simulink model "MIMO_Model_D_R1"  (R2013a)
settings: Solver=ode45  StartTime=0.0  StopTime=sim_length  MaxStep=1e-4  RelTol=1e-3
values from neighbouring files (symbols this model uses):
  A_d = sys_d.a    [MIMO_Controller.m]
  B_d = sys_d.b    [MIMO_Controller.m]
  C_d = sys_d.c    [MIMO_Controller.m]
  G_MIMO_d = place(A_d',C_d',P)'    [MIMO_Controller.m]
  K_MIMO_d = K_MIMO_Reg    [MIMO_Controller.m]
  omega_0 = 500    [MIMO_Controller.m]
  omega_Lim = -inf*(0-F_yIntercept)/Kf    [MIMO_Controller.m]
  Phi_IC = (0/180)*pi    (= 0)    [MIMO_Controller.m]
  Pitch_Setpoint = 0    [MIMO_Controller.m]
  Psi_IC = (0/180)*pi    (= 0)    [MIMO_Controller.m]
  PWM_LimHigher = 2*inf    (= inf)    [MIMO_Controller.m]
  PWM_LimLower = 1.1*-inf    (= -inf)    [MIMO_Controller.m]
  Theta_IC = (5/180)*pi    (= 0.0872664625997)    [MIMO_Controller.m]
  Ts = 30e-3    (= 0.03)    [MIMO_Controller.m]
  Yaw_Setpoint = 0    [MIMO_Controller.m]
undefined symbols (not defined in the file or in its folder): Drag, F_yIntercept, g, I_Phi, I_Psi, I_Theta, J, Kf, Kw, L, Mass, Motor_TimeConstant, Speed_yIntercept
libraries: simulink x6
settings Model: Creator=Ross  LastModifiedBy=Ross

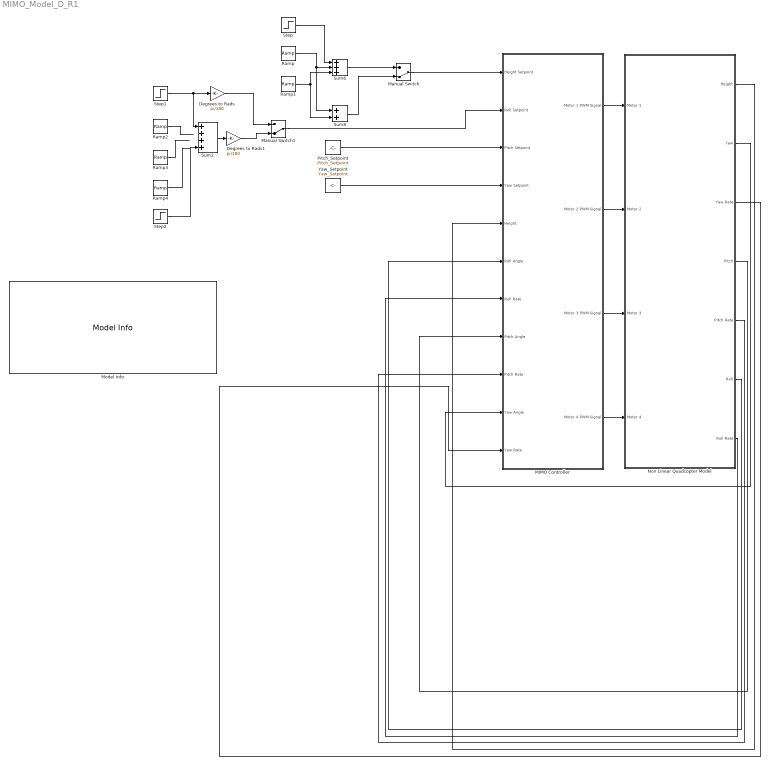
== system MIMO_Model_D_R1 ==
  Degrees to Rads : Gain  Gain=pi/180
  Degrees to Rads1 : Gain  Gain=pi/180
  MIMO Controller : Subsystem
  Manual Switch : ManualSwitch  CurrentSetting=0
  Manual Switch1 : ManualSwitch  CurrentSetting=0
  Model Info : simulink/Model-Wide Utilities/Model Info  InitialBlockCM=None  BlockCM=None  Frame=on  DisplayStringWithTags=|  HorizontalTextAlignment=Center  LeftAlignmentValue=0.5  SourceBlockDiagram=MIMO_Model_D_R1  TagMaxNumber=20
      | %<ModelName>
      | Simulink Diagram Used in Testing of Controllers designed for Quadcopters
      | Model version is %<ModelVersion>
      | 
      | %<Created>
      | %<ModifiedBy>
      | %<ModifiedDate>
      | %<ModifiedComment>
      | 
      | 
      | %<LastModifiedBy>
      | %<LastModificationDate>
      | %<Description>
  Non Linear Quadcopter Model : Subsystem
  "Pitch_Setpoint " : Constant  Value=Pitch_Setpoint
  Ramp : simulink/Sources/Ramp  slope=1  start=2  X0=0
  Ramp1 : simulink/Sources/Ramp  slope=-1  start=5  X0=0
  Ramp2 : simulink/Sources/Ramp  slope=10  start=2  X0=Ts
  Ramp3 : simulink/Sources/Ramp  slope=-20  start=4  X0=Ts
  Ramp4 : simulink/Sources/Ramp  slope=10  start=6  X0=Ts
  Step : Step  Time=10  SampleTime=0
  Step1 : Step  Time=2  After=20  SampleTime=Ts
  Step2 : Step  Time=4  After=-20  SampleTime=Ts
  Sum2 : Sum  Inputs=++++
  Sum6 : Sum  Inputs=+++  SampleTime=Ts
  Sum8 : Sum  SampleTime=Ts
  Yaw_Setpoint : Constant  Value=Yaw_Setpoint
  wires:
  Non Linear Quadcopter Model/1(Height) -> MIMO Controller/5(Height)
  Non Linear Quadcopter Model/5(Pitch Rate) -> MIMO Controller/9(Pitch Rate)
  Non Linear Quadcopter Model/7(Roll Rate) -> MIMO Controller/7(Roll Rate)
  Ramp/1 -> Sum8/1, Sum6/2
  Ramp1/1 -> Sum8/2, Sum6/3
  Step/1 -> Sum6/1
  Manual Switch/1 -> MIMO Controller/1(Height Setpoint)
  Sum8/1 -> Manual Switch/2
  Sum6/1 -> Manual Switch/1
  Non Linear Quadcopter Model/6(Roll) -> MIMO Controller/6(Roll Angle)
  Non Linear Quadcopter Model/4(Pitch) -> MIMO Controller/8(Pitch Angle)
  Ramp2/1 -> ?
  Ramp3/1 -> ?
  Step1/1 -> Sum2/1, Degrees to Rads/1
  Sum2/1 -> Degrees to Rads1/1
  Degrees to Rads/1 -> Manual Switch1/1
  "Pitch_Setpoint "/1 -> MIMO Controller/3(Pitch Setpoint)
  Manual Switch1/1 -> MIMO Controller/2(Roll Setpoint)
  Yaw_Setpoint/1 -> MIMO Controller/4(Yaw Setpoint)
  MIMO Controller/3(Motor 3 PWM Signal) -> Non Linear Quadcopter Model/3(Motor 3)
  MIMO Controller/2(Motor 2 PWM Signal) -> Non Linear Quadcopter Model/2(Motor 2)
  MIMO Controller/1(Motor 1 PWM Signal) -> Non Linear Quadcopter Model/1(Motor 1)
  Degrees to Rads1/1 -> Manual Switch1/2
  Step2/1 -> Sum2/4
  Ramp4/1 -> ?
  MIMO Controller/4(Motor 4 PWM Signal) -> Non Linear Quadcopter Model/4(Motor 4)
  Non Linear Quadcopter Model/2(Yaw) -> MIMO Controller/10(Yaw Angle)
  Non Linear Quadcopter Model/3(Yaw Rate) -> MIMO Controller/11(Yaw Rate)

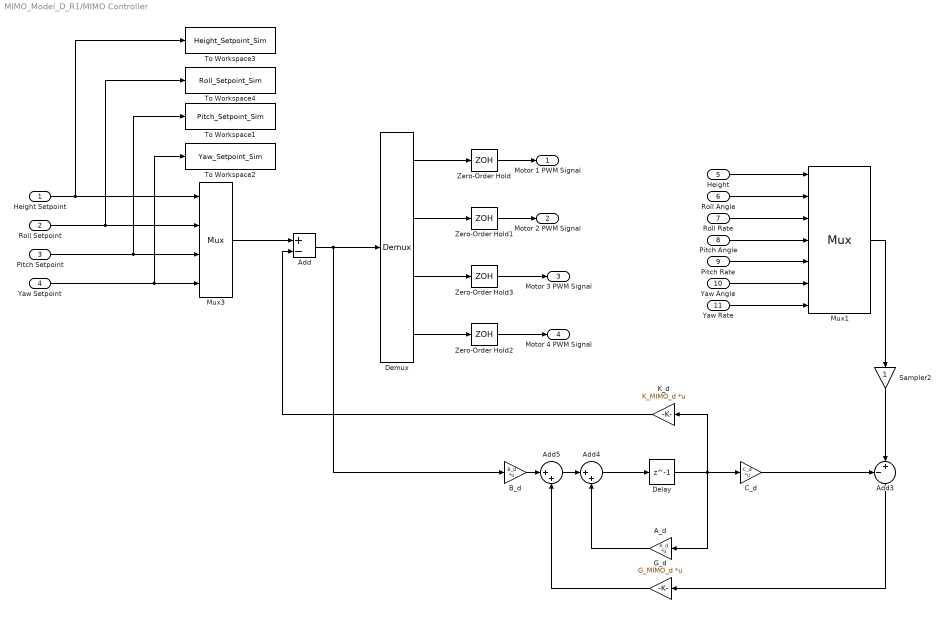
== system MIMO_Model_D_R1/MIMO Controller ==
  Height Setpoint : Inport
  Roll Setpoint : Inport  Port=2
  Pitch Setpoint : Inport  Port=3
  Yaw Setpoint : Inport  Port=4
  Height : Inport  Port=5
  Roll Angle : Inport  Port=6
  Roll Rate : Inport  Port=7
  Pitch Angle : Inport  Port=8
  Pitch Rate : Inport  Port=9
  Yaw Angle : Inport  Port=10
  Yaw Rate : Inport  Port=11
  A_d : Gain  Gain=A_d  Multiplication=Matrix(K*u)  SampleTime=Ts
  Add : Sum  Inputs=+-  SampleTime=Ts
  Add3 : Sum  Inputs=-+|
  Add4 : Sum  Inputs=|++
  Add5 : Sum  Inputs=|++
  "B_d " : Gain  Gain=B_d  Multiplication=Matrix(K*u)  SampleTime=Ts
  "C_d " : Gain  Gain=C_d  Multiplication=Matrix(K*u)  SampleTime=Ts
  Delay : Delay  DelayLength=1  InitialCondition=0  SampleTime=Ts
  Demux : Demux
  G_d : Gain  Gain=G_MIMO_d  Multiplication=Matrix(K*u)  SampleTime=Ts
  K_d : Gain  Gain=K_MIMO_d  Multiplication=Matrix(K*u)  SampleTime=Ts
  Mux1 : Mux  Inputs=7
      settings: DisplayOption=signals
  Mux3 : Mux
      settings: DisplayOption=signals
  Sampler2 : Gain  SampleTime=Ts
  To Workspace1 : ToWorkspace  VariableName=Pitch_Setpoint_Sim  SampleTime=-1  SaveFormat=Timeseries
  To Workspace2 : ToWorkspace  VariableName=Yaw_Setpoint_Sim  SampleTime=-1  SaveFormat=Timeseries
  To Workspace3 : ToWorkspace  VariableName=Height_Setpoint_Sim  SampleTime=-1  SaveFormat=Timeseries
  To Workspace4 : ToWorkspace  VariableName=Roll_Setpoint_Sim  SampleTime=-1  SaveFormat=Timeseries
  Zero-Order Hold{,1..3} (4 alike) : ZeroOrderHold  SampleTime=Ts
  Motor 1 PWM Signal : Outport
  Motor 2 PWM Signal : Outport  Port=2
  Motor 3 PWM Signal : Outport  Port=3
  Motor 4 PWM Signal : Outport  Port=4
  wires:
  Roll Angle/1 -> Mux1/2
  Height/1 -> Mux1/1
  Add5/1 -> Add4/1
  Mux1/1 -> Sampler2/1
  G_d/1 -> Add5/2
  A_d/1 -> Add4/2
  Add4/1 -> Delay/1
  "C_d "/1 -> Add3/1
  K_d/1 -> Add/2
  Sampler2/1 -> Add3/2
  "B_d "/1 -> Add5/1
  Delay/1 -> K_d/1, "C_d "/1, A_d/1
  Add3/1 -> G_d/1
  Add/1 -> "B_d "/1, Demux/1
  Roll Rate/1 -> Mux1/3
  Pitch Angle/1 -> Mux1/4
  Pitch Rate/1 -> Mux1/5
  Yaw Angle/1 -> Mux1/6
  Yaw Rate/1 -> Mux1/7
  Height Setpoint/1 -> To Workspace3/1, Mux3/1
  Roll Setpoint/1 -> To Workspace4/1, Mux3/2
  Pitch Setpoint/1 -> To Workspace1/1, Mux3/3
  Yaw Setpoint/1 -> To Workspace2/1, Mux3/4
  Mux3/1 -> Add/1
  Demux/1 -> Zero-Order Hold/1
  Demux/2 -> Zero-Order Hold1/1
  Demux/3 -> Zero-Order Hold3/1
  Demux/4 -> Zero-Order Hold2/1
  Zero-Order Hold/1 -> Motor 1 PWM Signal/1
  Zero-Order Hold1/1 -> Motor 2 PWM Signal/1
  Zero-Order Hold3/1 -> Motor 3 PWM Signal/1
  Zero-Order Hold2/1 -> Motor 4 PWM Signal/1

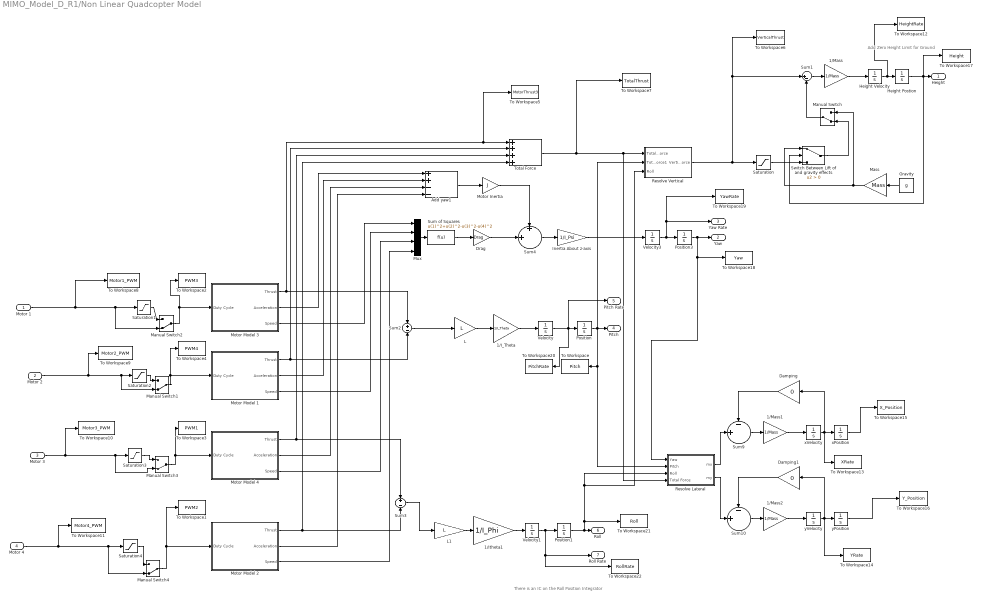
== system MIMO_Model_D_R1/Non Linear Quadcopter Model ==
  note: There is an IC on the Roll
      | Position Integrator
  note: Add Zero Height Limit
      | for Ground
  Motor 1 : Inport
  Motor 2 : Inport  Port=2
  Motor 3 : Inport  Port=3
  Motor 4 : Inport  Port=4
  1/I_Theta : Gain  Gain=1/I_Theta
  1/Itheta1 : Gain  Gain=1/I_Phi
  1/Mass : Gain  Gain=1/Mass
  1/Mass1 : Gain  Gain=1/Mass
  1/Mass2 : Gain  Gain=1/Mass
  Add yaw1 : Sum  Inputs=++--
  Damping : Gain  Gain=0
  Damping1 : Gain  Gain=0
  Drag : Gain  Gain=Drag
  Gravity : Constant  Value=g
  Height Postion : Integrator  LowerSaturationLimit=0
  Height Velocity : Integrator
  Inertia About z-axis : Gain  Gain=1/I_Psi
  L : Gain  Gain=L
  L1 : Gain  Gain=L
  Manual Switch{,1..4} (5 alike) : ManualSwitch  CurrentSetting=0
  Mass : Gain  Gain=Mass
  Motor Inertia : Gain  Gain=J
  Motor Model 1 : Subsystem
  Motor Model 2 : Subsystem
  Motor Model 3 : Subsystem
  Motor Model 4 : Subsystem
  Mux : Mux
  Position : Integrator  InitialCondition=Theta_IC
  Position1 : Integrator  InitialCondition=Phi_IC
  Position3 : Integrator  InitialCondition=Psi_IC
  Resolve Lateral : Subsystem
  Resolve Vertical : Subsystem
  Saturation : Saturate  UpperLimit=Mass*g  LowerLimit=-inf
  Saturation{1..4} (4 alike) : Saturate  UpperLimit=PWM_LimHigher  LowerLimit=PWM_LimLower
  Sum of Squares : Fcn  Expr=u(1)^2+u(2)^2-u(3)^2-u(4)^2
  Sum1 : Sum  Inputs=|+-
  Sum10 : Sum  Inputs=-|||+||||
  Sum2 : Sum  Inputs=+|-
  Sum3 : Sum  Inputs=+|-
  Sum4 : Sum  Inputs=+|||+||||
  Sum9 : Sum  Inputs=-|||+||||
  Switch Between Lift of and gravity effects : Switch  Criteria=u2 > Threshold
  To Workspace : ToWorkspace  VariableName=Pitch  SampleTime=-1  SaveFormat=Timeseries
  To Workspace1 : ToWorkspace  VariableName=PWM2  SampleTime=-1  SaveFormat=Timeseries
  To Workspace10 : ToWorkspace  VariableName=Motor3_PWM  SampleTime=-1  SaveFormat=Timeseries
  To Workspace11 : ToWorkspace  VariableName=Motor4_PWM  SampleTime=-1  SaveFormat=Timeseries
  To Workspace12 : ToWorkspace  VariableName=HeightRate  SampleTime=-1  SaveFormat=Timeseries
  To Workspace13 : ToWorkspace  VariableName=XRate  SampleTime=-1  SaveFormat=Timeseries
  To Workspace14 : ToWorkspace  VariableName=YRate  SampleTime=-1  SaveFormat=Timeseries
  To Workspace15 : ToWorkspace  VariableName=X_Position  SampleTime=-1  SaveFormat=Timeseries
  To Workspace16 : ToWorkspace  VariableName=Y_Position  SampleTime=-1  SaveFormat=Timeseries
  To Workspace17 : ToWorkspace  VariableName=Height  SampleTime=-1  SaveFormat=Timeseries
  To Workspace18 : ToWorkspace  VariableName=Yaw  SampleTime=-1  SaveFormat=Timeseries
  To Workspace19 : ToWorkspace  VariableName=YawRate  SampleTime=-1  SaveFormat=Timeseries
  To Workspace2 : ToWorkspace  VariableName=PWM3  SampleTime=-1  SaveFormat=Timeseries
  To Workspace20 : ToWorkspace  VariableName=PitchRate  SampleTime=-1  SaveFormat=Timeseries
  To Workspace21 : ToWorkspace  VariableName=Roll  SampleTime=-1  SaveFormat=Timeseries
  To Workspace22 : ToWorkspace  VariableName=RollRate  SampleTime=-1  SaveFormat=Timeseries
  To Workspace3 : ToWorkspace  VariableName=PWM1  SampleTime=-1  SaveFormat=Timeseries
  To Workspace4 : ToWorkspace  VariableName=PWM4  SampleTime=-1  SaveFormat=Timeseries
  To Workspace5 : ToWorkspace  VariableName=MotorThrust3  SampleTime=-1  SaveFormat=Timeseries
  To Workspace6 : ToWorkspace  VariableName=VerticalThrust  SampleTime=-1  SaveFormat=Timeseries
  To Workspace7 : ToWorkspace  VariableName=TotalThrust  SampleTime=-1  SaveFormat=Timeseries
  To Workspace8 : ToWorkspace  VariableName=Motor1_PWM  SampleTime=-1  SaveFormat=Timeseries
  To Workspace9 : ToWorkspace  VariableName=Motor2_PWM  SampleTime=-1  SaveFormat=Timeseries
  Total Force : Sum  Inputs=++++
  Velocity : Integrator
  Velocity1 : Integrator
  Velocity3 : Integrator
  xPosition : Integrator
  xVelocity : Integrator
  yPosition : Integrator
  yVelocity : Integrator
  Height : Outport
  Yaw : Outport  Port=2
  Yaw Rate : Outport  Port=3
  Pitch : Outport  Port=4
  Pitch Rate : Outport  Port=5
  Roll : Outport  Port=6
  Roll Rate : Outport  Port=7
  wires:
  Sum1/1 -> 1/Mass/1
  Motor 3/1 -> Manual Switch3/2, Saturation3/1, To Workspace10/1
  Add yaw1/1 -> Motor Inertia/1
  1/Mass/1 -> Height Velocity/1
  Motor Inertia/1 -> Sum4/1
  1/Mass1/1 -> xVelocity/1
  Sum9/1 -> 1/Mass1/1
  xPosition/1 -> To Workspace15/1
  Damping/1 -> Sum9/1
  xVelocity/1 -> To Workspace13/1, Damping/1, xPosition/1
  Motor Model 3/2(Acceleration) -> Add yaw1/1
  Height Velocity/1 -> To Workspace12/1, Height Postion/1
  Sum2/1 -> L/1
  1/I_Theta/1 -> Velocity/1
  Velocity/1 -> To Workspace20/1, Pitch Rate/1, Position/1
  Position/1 -> Resolve Vertical/2(Total Force1), Pitch/1, To Workspace/1, Resolve Lateral/2(Pitch)
  Total Force/1 -> To Workspace7/1, Resolve Lateral/4(Total Force), Resolve Vertical/1(Total Force)
  Sum of Squares/1 -> Drag/1
  Drag/1 -> Sum4/2
  Position3/1 -> To Workspace18/1, Resolve Lateral/1(Yaw), Yaw/1
  Velocity3/1 -> To Workspace19/1, Yaw Rate/1, Position3/1
  Inertia About z-axis/1 -> Velocity3/1
  Motor Model 2/1(Thrust) -> Total Force/4, Sum3/2
  L1/1 -> 1/Itheta1/1
  Velocity1/1 -> To Workspace22/1, Roll Rate/1, Position1/1
  Sum3/1 -> L1/1
  Position1/1 -> Roll/1, To Workspace21/1, Resolve Lateral/3(Roll), Resolve Vertical/3(Roll)
  1/Itheta1/1 -> Velocity1/1
  Motor Model 3/1(Thrust) -> To Workspace5/1, Total Force/1, Sum2/1
  Sum10/1 -> 1/Mass2/1
  1/Mass2/1 -> yVelocity/1
  Damping1/1 -> Sum10/1
  yVelocity/1 -> Damping1/1, To Workspace14/1, yPosition/1
  Height Postion/1 -> Switch Between Lift of and gravity effects/2, To Workspace17/1, Height/1
  Motor Model 4/2(Acceleration) -> Add yaw1/3
  Motor Model 1/1(Thrust) -> Total Force/2, Sum2/2
  Sum4/1 -> Inertia About z-axis/1
  Motor Model 4/1(Thrust) -> Total Force/3, Sum3/1
  Motor 1/1 -> To Workspace8/1, Manual Switch2/2, Saturation1/1
  Motor 2/1 -> Manual Switch1/2, Saturation2/1, To Workspace9/1
  Motor Model 1/2(Acceleration) -> Add yaw1/2
  Motor Model 2/2(Acceleration) -> Add yaw1/4
  Motor 4/1 -> Manual Switch4/2, Saturation4/1, To Workspace11/1
  Gravity/1 -> Mass/1
  Resolve Lateral/1(mx) -> Sum9/2
  Resolve Lateral/2(my) -> Sum10/2
  Motor Model 3/3(Speed) -> Mux/1
  Motor Model 1/3(Speed) -> Mux/2
  Motor Model 4/3(Speed) -> Mux/3
  Motor Model 2/3(Speed) -> Mux/4
  Mux/1 -> Sum of Squares/1
  L/1 -> 1/I_Theta/1
  Switch Between Lift of and gravity effects/1 -> Manual Switch/2
  Saturation/1 -> Switch Between Lift of and gravity effects/3
  Mass/1 -> Manual Switch/1, Switch Between Lift of and gravity effects/1
  Manual Switch/1 -> Sum1/2
  Resolve Vertical/1(Vertical Force) -> Sum1/1, To Workspace6/1, Saturation/1
  yPosition/1 -> To Workspace16/1
  Manual Switch2/1 -> To Workspace2/1, Motor Model 3/1(Duty Cycle)
  Manual Switch1/1 -> To Workspace4/1, Motor Model 1/1(Duty Cycle)
  Manual Switch3/1 -> Motor Model 4/1(Duty Cycle), To Workspace3/1
  Manual Switch4/1 -> To Workspace1/1, Motor Model 2/1(Duty Cycle)
  Saturation2/1 -> Manual Switch1/1
  Saturation4/1 -> Manual Switch4/1
  Saturation3/1 -> Manual Switch3/1
  Saturation1/1 -> Manual Switch2/1

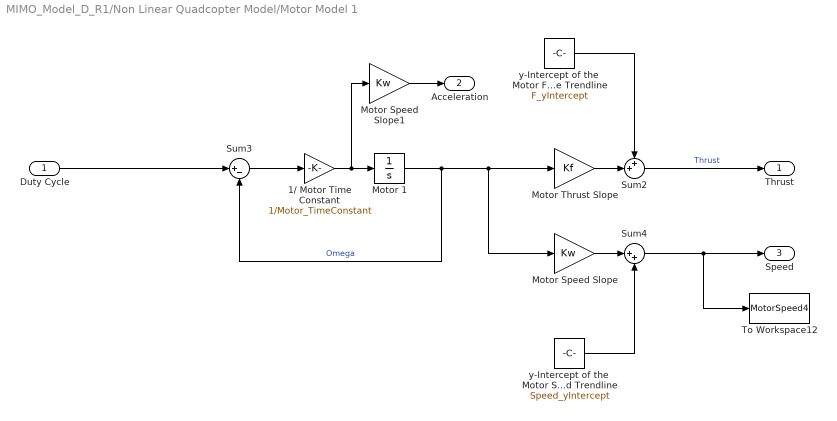
== system MIMO_Model_D_R1/Non Linear Quadcopter Model/Motor Model 1 ==
  Duty Cycle : Inport
  1/ Motor Time Constant : Gain  Gain=1/Motor_TimeConstant
  Motor 1 : Integrator  InitialCondition=omega_0  LimitOutput=on  LowerSaturationLimit=omega_Lim
  Motor Speed Slope : Gain  Gain=Kw
  Motor Speed Slope1 : Gain  Gain=Kw
  Motor Thrust Slope : Gain  Gain=Kf
  Sum2 : Sum  Inputs=++|
  Sum3 : Sum  Inputs=|+-
  Sum4 : Sum  Inputs=|++
  To Workspace12 : ToWorkspace  VariableName=MotorSpeed4  SampleTime=-1  SaveFormat=Timeseries
  y-Intercept of the  Motor Force Trendline : Constant  Value=F_yIntercept
  y-Intercept of the  Motor Speed Trendline : Constant  Value=Speed_yIntercept
  Thrust : Outport
  Acceleration : Outport  Port=2
  Speed : Outport  Port=3
  wires:
  Motor Thrust Slope/1 -> Sum2/2
  Motor 1/1 -> Sum3/2, Motor Speed Slope/1, Motor Thrust Slope/1  "Omega"
  Duty Cycle/1 -> Sum3/1
  Sum3/1 -> 1/ Motor Time Constant/1
  1/ Motor Time Constant/1 -> Motor 1/1, Motor Speed Slope1/1
  Motor Speed Slope/1 -> Sum4/1
  Motor Speed Slope1/1 -> Acceleration/1
  Sum2/1 -> Thrust/1  "Thrust"
  y-Intercept of the  Motor Force Trendline/1 -> Sum2/1
  y-Intercept of the  Motor Speed Trendline/1 -> Sum4/2
  Sum4/1 -> To Workspace12/1, Speed/1

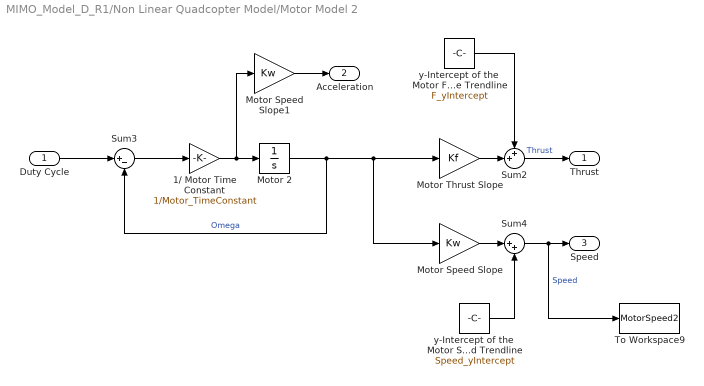
== system MIMO_Model_D_R1/Non Linear Quadcopter Model/Motor Model 2 ==
  Duty Cycle : Inport
  1/ Motor Time Constant : Gain  Gain=1/Motor_TimeConstant
  Motor 2 : Integrator  InitialCondition=omega_0  LimitOutput=on  LowerSaturationLimit=omega_Lim
  Motor Speed Slope : Gain  Gain=Kw
  Motor Speed Slope1 : Gain  Gain=Kw
  Motor Thrust Slope : Gain  Gain=Kf
  Sum2 : Sum  Inputs=++|
  Sum3 : Sum  Inputs=|+-
  Sum4 : Sum  Inputs=|++
  To Workspace9 : ToWorkspace  VariableName=MotorSpeed2  SampleTime=-1  SaveFormat=Timeseries
  y-Intercept of the  Motor Force Trendline : Constant  Value=F_yIntercept
  y-Intercept of the  Motor Speed Trendline : Constant  Value=Speed_yIntercept
  Thrust : Outport
  Acceleration : Outport  Port=2
  Speed : Outport  Port=3
  wires:
  Motor Thrust Slope/1 -> Sum2/2
  Motor 2/1 -> Sum3/2, Motor Speed Slope/1, Motor Thrust Slope/1  "Omega"
  Duty Cycle/1 -> Sum3/1
  Sum3/1 -> 1/ Motor Time Constant/1
  1/ Motor Time Constant/1 -> Motor 2/1, Motor Speed Slope1/1
  Motor Speed Slope/1 -> Sum4/1
  Motor Speed Slope1/1 -> Acceleration/1
  Sum2/1 -> Thrust/1  "Thrust"
  y-Intercept of the  Motor Force Trendline/1 -> Sum2/1
  Sum4/1 -> To Workspace9/1, Speed/1  "Speed"
  y-Intercept of the  Motor Speed Trendline/1 -> Sum4/2

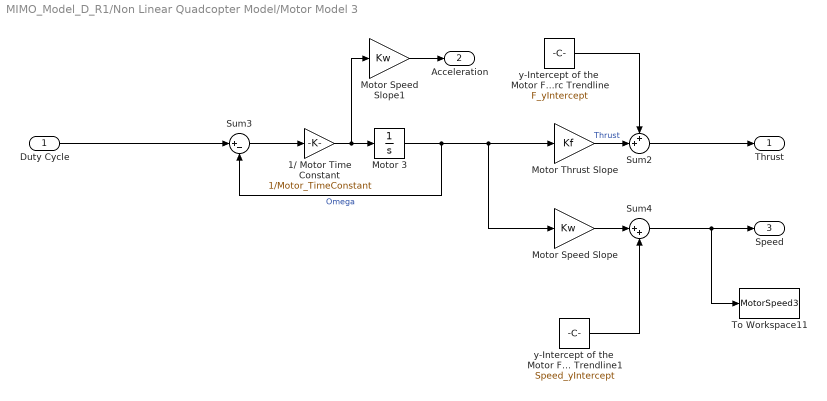
== system MIMO_Model_D_R1/Non Linear Quadcopter Model/Motor Model 3 ==
  Duty Cycle : Inport
  1/ Motor Time Constant : Gain  Gain=1/Motor_TimeConstant
  Motor 3 : Integrator  InitialCondition=omega_0  LimitOutput=on  LowerSaturationLimit=omega_Lim
  Motor Speed Slope : Gain  Gain=Kw
  Motor Speed Slope1 : Gain  Gain=Kw
  Motor Thrust Slope : Gain  Gain=Kf
  Sum2 : Sum  Inputs=++|
  Sum3 : Sum  Inputs=|+-
  Sum4 : Sum  Inputs=|++
  To Workspace11 : ToWorkspace  VariableName=MotorSpeed3  SampleTime=-1  SaveFormat=Timeseries
  y-Intercept of the  Motor Forc Trendline : Constant  Value=F_yIntercept
  y-Intercept of the  Motor Forc Trendline1 : Constant  Value=Speed_yIntercept
  Thrust : Outport
  Acceleration : Outport  Port=2
  Speed : Outport  Port=3
  wires:
  Motor Thrust Slope/1 -> Sum2/2  "Thrust"
  Motor 3/1 -> Sum3/2, Motor Speed Slope/1, Motor Thrust Slope/1  "Omega"
  Duty Cycle/1 -> Sum3/1
  Sum3/1 -> 1/ Motor Time Constant/1
  1/ Motor Time Constant/1 -> Motor 3/1, Motor Speed Slope1/1
  Motor Speed Slope/1 -> Sum4/1
  Motor Speed Slope1/1 -> Acceleration/1
  y-Intercept of the  Motor Forc Trendline/1 -> Sum2/1
  y-Intercept of the  Motor Forc Trendline1/1 -> Sum4/2
  Sum2/1 -> Thrust/1
  Sum4/1 -> To Workspace11/1, Speed/1

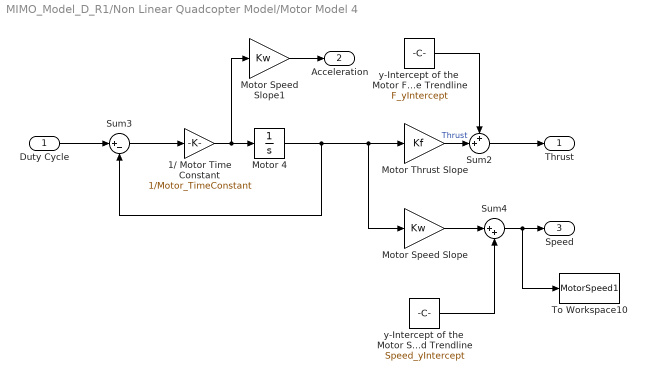
== system MIMO_Model_D_R1/Non Linear Quadcopter Model/Motor Model 4 ==
  Duty Cycle : Inport
  1/ Motor Time Constant : Gain  Gain=1/Motor_TimeConstant
  Motor 4 : Integrator  InitialCondition=omega_0  LimitOutput=on  LowerSaturationLimit=omega_Lim
  Motor Speed Slope : Gain  Gain=Kw
  Motor Speed Slope1 : Gain  Gain=Kw
  Motor Thrust Slope : Gain  Gain=Kf
  Sum2 : Sum  Inputs=++|
  Sum3 : Sum  Inputs=|+-
  Sum4 : Sum  Inputs=|++
  To Workspace10 : ToWorkspace  VariableName=MotorSpeed1  SampleTime=-1  SaveFormat=Timeseries
  y-Intercept of the  Motor Force Trendline : Constant  Value=F_yIntercept
  y-Intercept of the  Motor Speed Trendline : Constant  Value=Speed_yIntercept
  Thrust : Outport
  Acceleration : Outport  Port=2
  Speed : Outport  Port=3
  wires:
  Motor Thrust Slope/1 -> Sum2/2  "Thrust"
  Motor 4/1 -> Sum3/2, Motor Speed Slope/1, Motor Thrust Slope/1
  Duty Cycle/1 -> Sum3/1
  Sum3/1 -> 1/ Motor Time Constant/1
  1/ Motor Time Constant/1 -> Motor 4/1, Motor Speed Slope1/1
  Motor Speed Slope/1 -> Sum4/1
  Motor Speed Slope1/1 -> Acceleration/1
  Sum2/1 -> Thrust/1
  y-Intercept of the  Motor Force Trendline/1 -> Sum2/1
  Sum4/1 -> To Workspace10/1, Speed/1
  y-Intercept of the  Motor Speed Trendline/1 -> Sum4/2

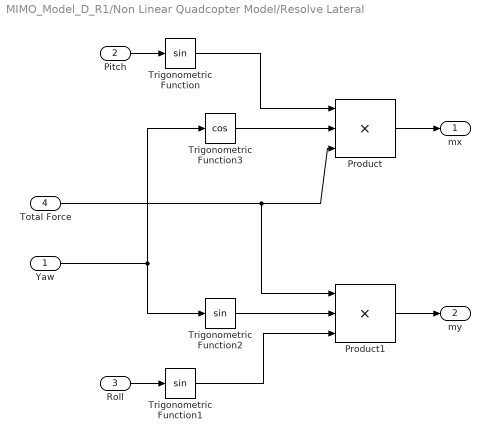
== system MIMO_Model_D_R1/Non Linear Quadcopter Model/Resolve Lateral ==
  Yaw : Inport
  Pitch : Inport  Port=2
  Roll : Inport  Port=3
  Total Force : Inport  Port=4
  Product : Product  Inputs=3
  Product1 : Product  Inputs=3
  Trigonometric Function : Trigonometry
  Trigonometric Function1 : Trigonometry
  Trigonometric Function2 : Trigonometry
  Trigonometric Function3 : Trigonometry  Operator=cos
  mx : Outport
  my : Outport  Port=2
  wires:
  Trigonometric Function/1 -> Product/1
  Total Force/1 -> Product1/1, Product/3
  Product/1 -> mx/1
  Roll/1 -> Trigonometric Function1/1
  Trigonometric Function1/1 -> Product1/3
  Product1/1 -> my/1
  Trigonometric Function3/1 -> Product/2
  Trigonometric Function2/1 -> Product1/2
  Yaw/1 -> Trigonometric Function2/1, Trigonometric Function3/1
  Pitch/1 -> Trigonometric Function/1

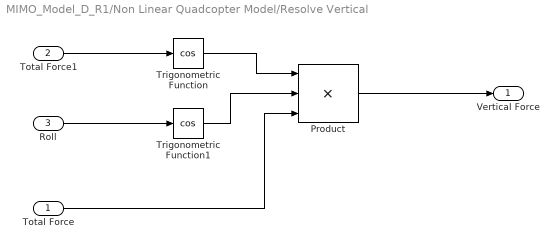
== system MIMO_Model_D_R1/Non Linear Quadcopter Model/Resolve Vertical ==
  Total Force : Inport
  Total Force1 : Inport  Port=2
  Roll : Inport  Port=3
  Product : Product  Inputs=3
  Trigonometric Function : Trigonometry  Operator=cos
  Trigonometric Function1 : Trigonometry  Operator=cos
  Vertical Force : Outport
  wires:
  Trigonometric Function/1 -> Product/1
  Total Force/1 -> Product/3
  Roll/1 -> Trigonometric Function1/1
  Total Force1/1 -> Trigonometric Function/1
  Product/1 -> Vertical Force/1
  Trigonometric Function1/1 -> Product/2
